simulink model "scd3busMicrogridDroopControlFidelityLevels3Inv"  (R2025b)
settings: Solver=ode15s  StartTime=0.0  StopTime=24  RelTol=1e-3
PreLoadFcn:
  | scd3busMicrogridDroopControlDataFidelityLevels3Inv;
  | 
  | %% Controller variants
  | % Create variant controls for converter controller. Controller has two
  | % different levels of fidelity: Averaged, AveragedPulse, Pulse
  | Averaged = Simulink.VariantExpression;
  | Averaged.Condition = 'fidelity==scd3busMicrogridDroopControl_variants_enum.Low';
  | Pulse = Simulink.VariantExpression;
  | Pulse.Condition = 'fidelity==scd3busMicrogridDroopControl_variants_enum.High';
  | 
  | %% Plant variants
  | % Create variant controls for converter plant. Plant has three different
  | % levels of fidelity.
  | AveragedNonSwitch = Simulink.VariantExpression;
  | AveragedNonSwitch.Condition = 'fidelity==scd3busMicrogridDroopControl_variants_enum.Low';
  | PulseSwitch = Simulink.VariantExpression;
  | PulseSwitch.Condition = 'fidelity==scd3busMicrogridDroopControl_variants_enum.High';
  | 
  | %% Set up variables ready for simulation
  | fidelity = scd3busMicrogridDroopControl_variants_enum.High;
  | Ts = 5e-6;
  | Ts_V = 1e-6;
  | Tsc = 1e-4;
  | Tsc_V = 5e-4;
values from neighbouring files (symbols this model uses):
  consensus_enable = 1    [scd3busMicrogridDroopControlDataFidelityLevels3Inv.m]
  fgrid = 60    [scd3busMicrogridDroopControlDataFidelityLevels.m]    (also in scd3busMicrogridDroopControlDataFidelityLevels3Inv.m)
  Kdroop_fp1 = 0.03/2    (= 0.015)    [scd3busMicrogridDroopControlDataFidelityLevels3Inv.m]
  Kdroop_fp2 = 0.03/2    (= 0.015)    [scd3busMicrogridDroopControlDataFidelityLevels3Inv.m]
  Kdroop_vq1 = 0.05/2    (= 0.025)    [scd3busMicrogridDroopControlDataFidelityLevels3Inv.m]
  Kdroop_vq2 = 0.05/2    (= 0.025)    [scd3busMicrogridDroopControlDataFidelityLevels3Inv.m]
  Ki_vd = 850    [scd3busMicrogridDroopControlDataFidelityLevels.m]    (also in scd3busMicrogridDroopControlDataFidelityLevels3Inv.m)
  Ki_vq = 850    [scd3busMicrogridDroopControlDataFidelityLevels.m]    (also in scd3busMicrogridDroopControlDataFidelityLevels3Inv.m)
  Kp_vd = 0.36    [scd3busMicrogridDroopControlDataFidelityLevels.m]    (also in scd3busMicrogridDroopControlDataFidelityLevels3Inv.m)
  Kp_vq = 0.36    [scd3busMicrogridDroopControlDataFidelityLevels.m]    (also in scd3busMicrogridDroopControlDataFidelityLevels3Inv.m)
  Vdc1 = 1000    [scd3busMicrogridDroopControlDataFidelityLevels.m]    (also in scd3busMicrogridDroopControlDataFidelityLevels3Inv.m)
  Vdc2 = 1000    [scd3busMicrogridDroopControlDataFidelityLevels.m]    (also in scd3busMicrogridDroopControlDataFidelityLevels3Inv.m)
  Vrms = 380    [scd3busMicrogridDroopControlDataFidelityLevels.m]    (also in scd3busMicrogridDroopControlDataFidelityLevels3Inv.m)
undefined symbols (not defined in the file or in its folder): DiscIntNeverNeededParam
libraries: ee_lib x29, nesl_utility x27, fl_lib x15, eeTransforms x4, eeSinusoidalMeasurement x4, slpidlib x4, eePwmGeneratorTwoLevel x2, eePowerMeasurement x2, simulink x2, SignalEditorBlockLib x1
(part 2 of 3)

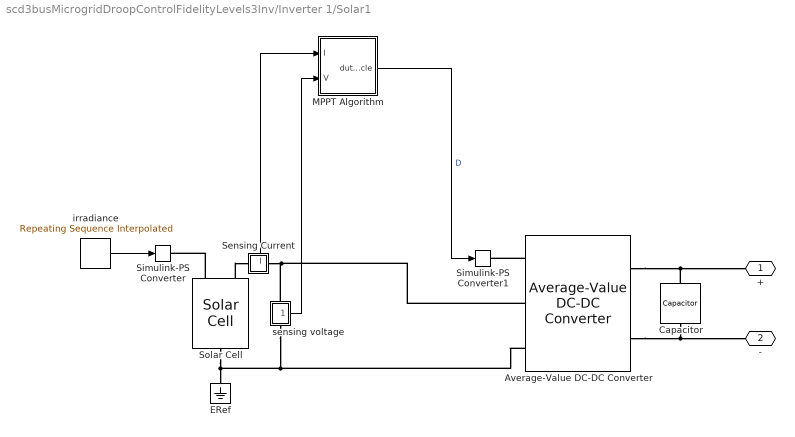
== system scd3busMicrogridDroopControlFidelityLevels3Inv/Inverter 1/Solar1 ==
  Average-Value DC-DC Converter : ee_lib/Semiconductors & Converters/Converters/Average-Value DC-DC Converter  implementation_option=ee.enum.converters.implementation.behavioral  converter_type=ee.enum.converters.dcdctype.boost  control_option=ee.enum.converters.controlinput.dutycycle  efficiency_option=ee.enum.converters.efficiency.constant  efficiency_fixed=100  i_vec=[0, 2, 5] A  efficiency_vec=[90, 95, 98]  Lf=1e-6 H  Rl=0 Ohm  Cf=1e-7 F  Rc=1e-6 Ohm  iL_specify=off  iL_priority=High  iL=0 A  iL_nominal_specify=off  iL_nominal_value=1  iL_nominal_unit=A  vc_specify=off  vc_priority=High  vc=0 V  vc_nominal_specify=off  vc_nominal_value=1  vc_nominal_unit=V
      settings: InternalSimscapePortConfiguration="{\"Bottom\":[],\"Left\":[{\"id\":\"DutyCycle\",\"label\":\"DutyCycle\",\"type\":\"input\"},{\"id\":\"p1\",\"label\":\"1+\",\"type\":\"foundation.electrical.electrical\"},{\"id\":\"n1\",\"label\":\"1-\",\"type\":\"foundation.electrical.electrical\"}],\"Right\":[{\"id\":\"p2\",\"label\":\"2+\",\"type\":\"foundation.electrical.electrical\"},{\"id\":\"n2\",\"label\":\"2-\",\"type\":\"foundation.electrical.electrical\"}],\"Top\":[]}"
  Capacitor : fl_lib/Electrical/Electrical Elements/Capacitor  c=10 mF  r=1e-6 Ohm  g=0 1/Ohm  i_specify=off  i_priority=None  i=0 A  i_nominal_specify=off  i_nominal_value=1  i_nominal_unit=A  v_specify=off  v_priority=None  v=0 V  v_nominal_specify=off  v_nominal_value=1  v_nominal_unit=V  vc_specify=off  vc_priority=High  vc=1000 V  vc_nominal_specify=off  vc_nominal_value=1  vc_nominal_unit=V
  ERef : fl_lib/Electrical/Electrical Elements/Electrical Reference
  MPPT Algorithm : Subsystem
  Sensing Current : Subsystem
      settings: PortSchema="{\"entries\":[{\"content\":{\"sides\":[{\"content\":{\"connectorIds\":[\"LConn1\"]},\"type\":\"ConnectorPlacement.EquallySpacedRectSide\",\"uuid\":\"08eaf192-3836-4d70-9f6a-c3aee0977ea6\"},{\"content\":{\"connectorIds\":[\"RConn1\"],\"side\":\"RIGHT\"},\"type\":\"ConnectorPlacement.EquallySpacedRectSide\",\"uuid\":\"69615d36-c1bf-4d31-b3e4-77c73286e7c7\"},{\"content\":{\"connectorIds\":[\"Out1\"],\"side\":\"TOP\"},\"type\":\"ConnectorPlacement.EquallySpacedRectSide\",\"uuid\":\"21e31d90-f675-47e5-98f5-1bf7e6a5fdbe\"}]},\"type\":\"ConnectorPlacement.EquallySpacedConnector\",\"uuid\":\"068abd2e-abc9-41d7-b40e-d83d3e3b9346\"}],\"packageUris\":[\"http://schema.mathworks.com/mf0/Connector/R2020b\"],\"version\":\"1.0\"}"
      mask Display: disp('i')
  Simulink-PS Converter : nesl_utility/Simulink-PS Converter  PhysicalDomain=network_engine_domain  SubClassName=ps_input  LeftPortType=input  RightPortType=output  PseudoPeriodic=off  Frequencies=[]  NoiseDistribution=none  NoiseParameters=[]  Unit=1  AffineConversion=off  FilteringAndDerivatives=provide  SimscapeFilterOrder=1  InputFilterTimeConstant=0.001  UdotUserProvided=0
  Simulink-PS Converter1 : nesl_utility/Simulink-PS Converter  PhysicalDomain=network_engine_domain  SubClassName=ps_input  LeftPortType=input  RightPortType=output  PseudoPeriodic=off  Frequencies=[]  NoiseDistribution=none  NoiseParameters=[]  Unit=1  AffineConversion=off  FilteringAndDerivatives=provide  SimscapeFilterOrder=1  InputFilterTimeConstant=0.001  UdotUserProvided=0
  Solar Cell : ee_lib/Sources/Solar Cell  prm=3  Isc=10.14 A  Voc=0.67 V  Is=3.24823447983853e-07 A  Is2=9.37081970792037e-10 A  Iph=10.140005507508 A  Ir0=1000 W/m^2  ec=1.51118472243322  N2=2.60259908345858  Rs=1.94548269975201e-05 Ohm  Rp=682.95993142779 Ohm  N_series=60 * 30  N_parallel=8  TIPH1=0.000499942933005141 1/K  EG=1.12 eV  TXIS1=4.23641510120988  TXIS2=16.2689137700667  TRS1=0.243341028305912  TRP1=0 % Parameter not set  Tmeas=25 degC  TFIXED=25 degC  thermal_mass=100 % Parameter not set J/K  initial_temperature=25 degC
  "irradiance " : simulink/Sources/Repeating Sequence Interpolated  OutValues=[5 5 5 5 5 5 5 5 5 5 5 5 5 5 5 5 5 5 5 5 5 5 5 5]*200  TimeValues=[0 1 2 3 4 5 6 7 8 9 10 11 12 13 14 15 16 17 18 19 20 21 22 23]  LookUpMeth=Interpolation-Use End Values  tsamp=Ts_DC  OutMin=[]  OutMax=[]  OutDataTypeStr=double  OutputDataTypeScalingMode=double  OutDataType=fixdt(0,8)  OutScaling=2^-10
  sensing voltage : Subsystem
      settings: PortSchema="{\"entries\":[{\"content\":{\"sides\":[{\"content\":{\"connectorIds\":[\"LConn1\"]},\"type\":\"ConnectorPlacement.EquallySpacedRectSide\",\"uuid\":\"08eaf192-3836-4d70-9f6a-c3aee0977ea6\"},{\"content\":{\"connectorIds\":[\"RConn1\"],\"side\":\"RIGHT\"},\"type\":\"ConnectorPlacement.EquallySpacedRectSide\",\"uuid\":\"69615d36-c1bf-4d31-b3e4-77c73286e7c7\"},{\"content\":{\"connectorIds\":[],\"side\":\"TOP\"},\"type\":\"ConnectorPlacement.EquallySpacedRectSide\",\"uuid\":\"21e31d90-f675-47e5-98f5-1bf7e6a5fdbe\"},{\"content\":{\"connectorIds\":[\"Out1\"],\"side\":\"BOTTOM\"},\"type\":\"ConnectorPlacement.EquallySpacedRectSide\",\"uuid\":\"23a77980-6beb-4147-b48e-adf9e1983263\"}]},\"type\":\"ConnectorPlacement.EquallySpacedConnector\",\"uuid\":\"068abd2e-abc9-41d7-b40e-d83d3e3b9346\"}],\"packageUris\":[\"http://schema.mathworks.com/mf0/Connector/R2020b\"],\"version\":\"1.0\"}"
      mask Display: disp('v')
  + : PMIOPort  Side=Right
  - : PMIOPort  Port=2  Side=Right
  wires:
  "irradiance "/1 -> Simulink-PS Converter/1
  Sensing Current/1(I) -> MPPT Algorithm/1(I)
  sensing voltage/1(V) -> MPPT Algorithm/2(V)
  MPPT Algorithm/1(duty_cycle) -> Simulink-PS Converter1/1  "D"
  connections:
  Average-Value DC-DC Converter/LConn2 -- Sensing Current/RConn1 -- sensing voltage/LConn1
  Average-Value DC-DC Converter/LConn3 -- sensing voltage/RConn1 -- ERef/LConn1 -- Solar Cell/RConn1
  Average-Value DC-DC Converter/LConn1 -- Simulink-PS Converter1/RConn1
  Solar Cell/LConn1 -- Simulink-PS Converter/RConn1
  Solar Cell/LConn2 -- Sensing Current/LConn1
  Average-Value DC-DC Converter/RConn1 -- +/RConn1 -- Capacitor/LConn1
  Average-Value DC-DC Converter/RConn2 -- -/RConn1 -- Capacitor/RConn1

== system scd3busMicrogridDroopControlFidelityLevels3Inv/Inverter 2/Average-Value Signal1 ==
  ModWave : Inport
  Bias : Bias  Bias=1  SaturateOnIntegerOverflow=off
  Bias1 : Bias  Bias=1  SaturateOnIntegerOverflow=off
  Gain : Gain  Gain=-1
  Mod. Index1 : Gain  Gain=0.5
  Mux : Mux  Inputs=2
  Rate Transition : RateTransition  OutPortSampleTime=Ts_V
  Selector4 : Selector  InputPortWidth=6  IndexOptions=Index vector (dialog)  Indices=[1 4 2 5 3 6]  OutputSizes=1
  DutyCycle : Outport
  wires:
  ModWave/1 -> Rate Transition/1
  Gain/1 -> Bias1/1
  Mod. Index1/1 -> Gain/1, Mux/1
  Bias/1 -> Mod. Index1/1
  Rate Transition/1 -> Bias/1
  Selector4/1 -> DutyCycle/1
  Bias1/1 -> Mux/2
  Mux/1 -> Selector4/1

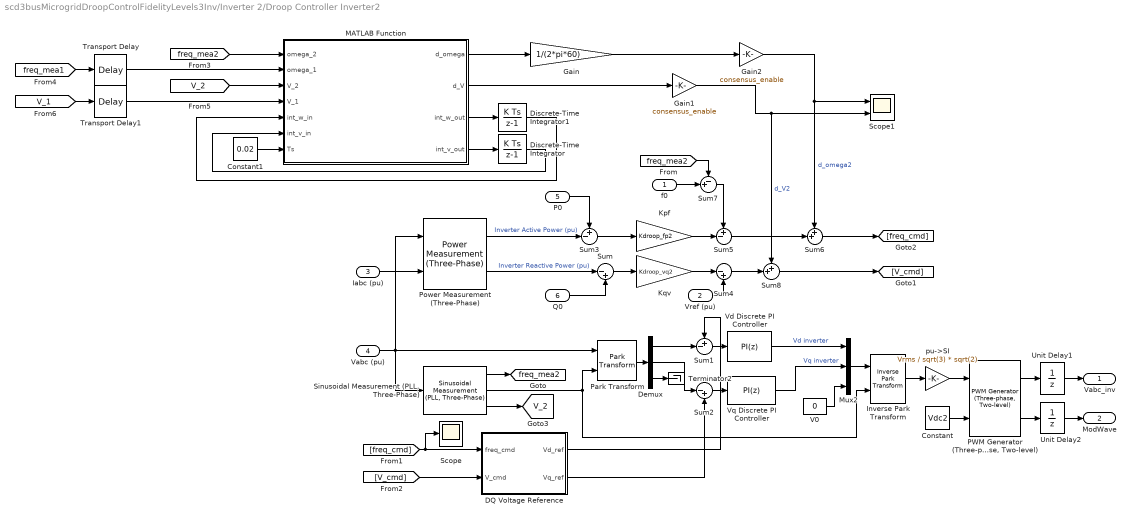
== system scd3busMicrogridDroopControlFidelityLevels3Inv/Inverter 2/Droop Controller Inverter2 ==
  f0 : Inport
  Vref (pu) : Inport  Port=2
  Iabc (pu) : Inport  Port=3
  Vabc (pu) : Inport  Port=4
  P0 : Inport  Port=5
  Q0 : Inport  Port=6
  Constant : Constant  Value=Vdc2
  Constant1 : Constant  Value=0.02
  DQ Voltage Reference : Subsystem
  Demux : Demux  Outputs=3
  Discrete-Time Integrator : DiscreteIntegrator  SampleTime=0.02  ICPrevOutput=DiscIntNeverNeededParam  ICPrevScaledInput=DiscIntNeverNeededParam
  Discrete-Time Integrator1 : DiscreteIntegrator  SampleTime=0.02  ICPrevOutput=DiscIntNeverNeededParam  ICPrevScaledInput=DiscIntNeverNeededParam
  Gain : Gain  Gain=1/(2*pi*60)
  Gain1 : Gain  Gain=consensus_enable
  Gain2 : Gain  Gain=consensus_enable
  Inverse Park Transform : eeTransforms/Inverse Park Transform  AxisAlignment=Q-axis  PowerInvariant=off
  Kpf : Gain  Gain=Kdroop_fp2
  Kqv : Gain  Gain=Kdroop_vq2
  MATLAB Function : MATLAB Function  TreatAsAtomicUnit=on
  Mux2 : Mux  Inputs=3
  "PWM Generator (Three-phase, Two-level)" : eePwmGeneratorTwoLevel/PWM Generator (Three-phase, Two-level)  PWMMode=Continuous PWM (CPWM)  CPWMMode=SPWM: sinusoidal PWM  DPWMMode=60 DPWM: 60 degree discontinuous PWM  fsw=fsw_V  Ts=Ts_V
  Park Transform : eeTransforms/Park Transform  AxisAlignment=Q-axis  PowerInvariant=off
  Power Measurement (Three-Phase) : eePowerMeasurement/Power Measurement (Three-Phase)  LabelModeActiveChoice=Discrete  F=fgrid  K=1  Seq=Positive  Ts=Ts
  Scope : Scope
      settings: ActiveDisplayYMinimum=-2.22443  ActiveDisplayYMaximum=1.7851
  Scope1 : Scope  NumInputPorts=2
      settings: ActiveDisplayYMinimum=-0.013262911924324612  ActiveDisplayYMaximum=0.013262911924324612
  "Sinusoidal Measurement (PLL, Three-Phase)" : eeSinusoidalMeasurement/Sinusoidal Measurement (PLL, Three-Phase)  Kp_LF=180  Ki_LF=3200  F0=fgrid  Theta0=0  Ts=Ts_V
  Sum : Sum  Inputs=|-+
  Sum1 : Sum  Inputs=+-|  InputSameDT=on  SaturateOnIntegerOverflow=on  OutDataTypeStr=Inherit: Same as first input
  Sum2 : Sum  Inputs=|-+  InputSameDT=on  SaturateOnIntegerOverflow=on  OutDataTypeStr=Inherit: Same as first input
  Sum3 : Sum  Inputs=+-|
  Sum4 : Sum  Inputs=|-+
  Sum5 : Sum  Inputs=+-|
  Sum6 : Sum  Inputs=++|
  Sum7 : Sum  Inputs=-+|
  Sum8 : Sum  Inputs=++|
  Terminator2 : Terminator
  Transport Delay : TransportDelay  DelayTime=0.1
  Transport Delay1 : TransportDelay  DelayTime=0.1
  Unit Delay1 : UnitDelay  SampleTime=Ts_V  HasFrameUpgradeWarning=on
  Unit Delay2 : UnitDelay  SampleTime=Ts_V  HasFrameUpgradeWarning=on
  V0 : Constant  Value=0
  Vd Discrete PI Controller : slpidlib/PID Controller  Controller=PI  Form=Parallel  TimeDomain=Discrete-time  UseExternalTs=off  SampleTime=Ts_V  IntegratorMethod=Forward Euler  FilterMethod=Forward Euler  ControllerParametersSource=internal  P=Kp_vd  I=Ki_vd  UseKiTs=off  D=0  UseExternalDerivativeSource=off  N=100  UseFilter=on  TunerSelectOption=Transfer Function Based (PID Tuner App)  InitialConditionSource=internal  InitialConditionForIntegrator=0.62  InitialConditionForFilter=0  DifferentiatorICPrevScaledInput=0  ExternalReset=none  TrackingMode=off  Kt=1  LimitOutput=on  SatLimitsSource=internal  UpperSaturationLimit=1  LowerSaturationLimit=0  LinearizeAsGain=on  AntiWindupMode=none  Kb=1  LimitIntegrator=off  UpperIntegratorSaturationLimit=inf  LowerIntegratorSaturationLimit=-inf  POutMin=[]  POutMax=[]  IOutMin=[]  IOutMax=[]  DOutMin=[]  DOutMax=[]  NOutMin=[]  NOutMax=[]  SumOutMin=[]  SumOutMax=[]  SaturationOutMin=[]  SaturationOutMax=[]  PParamMin=[]  PParamMax=[]  IParamMin=[]  IParamMax=[]  DParamMin=[]  DParamMax=[]  NParamMin=[]  NParamMax=[]  KbParamMin=[]  KbParamMax=[]  KtParamMin=[]  KtParamMax=[]  KbOutMin=[]  KbOutMax=[]  KtOutMin=[]  KtOutMax=[]  IntegratorOutMin=[]  IntegratorOutMax=[]  FilterOutMin=[]  FilterOutMax=[]  SumI1OutMin=[]  SumI1OutMax=[]  SumI2OutMin=[]  SumI2OutMax=[]  SumI3OutMin=[]  SumI3OutMax=[]  SumI4OutMin=[]  SumI4OutMax=[]  SumDOutMin=[]  SumDOutMax=[]  DifferentiatorOutMin=[]  DifferentiatorOutMax=[]  FilterDiffOutCoefMin=[]  FilterDiffOutCoefMax=[]  ReciprocalOutMin=[]  ReciprocalOutMax=[]  SumDenOutMin=[]  SumDenOutMax=[]  SumNumOutMin=[]  SumNumOutMax=[]  DivideOutMin=[]  DivideOutMax=[]  UdiffTsProdOutMin=[]  UdiffTsProdOutMax=[]  NTsProdOutMin=[]  NTsProdOutMax=[]  UintegralTsProdOutMin=[]  UintegralTsProdOutMax=[]  UngainTsProdOutMin=[]  UngainTsProdOutMax=[]  ClampingZeroOutDataTypeStr=Inherit: Inherit via back propagation  ClampingZeroOutMin=[]  ClampingZeroOutMax=[]  FilterDenConstantOutDataTypeStr=Inherit: Inherit via back propagation  FilterDenConstantOutMin=[]  FilterDenConstantOutMax=[]  PCopyOutDataTypeStr=Inherit: Inherit via back propagation  PCopyOutMin=[]  PCopyOutMax=[]  NCopyOutDataTypeStr=Inherit: Inherit via back propagation  NCopyOutMin=[]  NCopyOutMax=[]  IntegratorContinuousStateAttributes=''  IntegratorStateMustResolveToSignalObject=off  IntegratorRTWStateStorageClass=Auto  FilterContinuousStateAttributes=''  FilterStateMustResolveToSignalObject=off  FilterRTWStateStorageClass=Auto  ParallelPVariant=InternalParameters  IdealPVariant=Disabled  IVariant=InternalParameters  DVariant=Disabled  IntegratorVariant=Discrete  SatVariant=Enabled  AWVariant=Passthrough  PCopyVariant=Disabled  TRVariant=Disabled  FdbkBlocksVariant=Forward  IdealPFdbkVariant=Disabled  SatFdbkVariant=Disabled  DerivativeFilterVariant=Disabled  NVariant=Disabled  NCopyVariant=Disabled_SignalSpec  FilterICVariant=Disabled  IntegratorICVariant=InternalICs  ExternalResetVariant=Disabled  TRSumVariant=Passthrough  SumFdbkVariant=Disabled  SumVariant=Sum_PI  TsampFilterVariant=InternalTs  TsampNgainVariant=Passthrough  TsampIntegralVariant=Disabled_SignalSpec  ExternalSaturationOutDataTypeStr=Inherit: Same as second input  DerivativeSourceVariant=Disabled  PreIntVariant=InternalPreInt
  Vq Discrete PI Controller : slpidlib/PID Controller  Controller=PI  Form=Parallel  TimeDomain=Discrete-time  UseExternalTs=off  SampleTime=Ts_V  IntegratorMethod=Forward Euler  FilterMethod=Forward Euler  ControllerParametersSource=internal  P=Kp_vq  I=Ki_vq  UseKiTs=off  D=0  UseExternalDerivativeSource=off  N=100  UseFilter=on  TunerSelectOption=Transfer Function Based (PID Tuner App)  InitialConditionSource=internal  InitialConditionForIntegrator=0  InitialConditionForFilter=0  DifferentiatorICPrevScaledInput=0  ExternalReset=none  TrackingMode=off  Kt=1  LimitOutput=on  SatLimitsSource=internal  UpperSaturationLimit=1  LowerSaturationLimit=0  LinearizeAsGain=on  AntiWindupMode=none  Kb=1  LimitIntegrator=off  UpperIntegratorSaturationLimit=inf  LowerIntegratorSaturationLimit=-inf  POutMin=[]  POutMax=[]  IOutMin=[]  IOutMax=[]  DOutMin=[]  DOutMax=[]  NOutMin=[]  NOutMax=[]  SumOutMin=[]  SumOutMax=[]  SaturationOutMin=[]  SaturationOutMax=[]  PParamMin=[]  PParamMax=[]  IParamMin=[]  IParamMax=[]  DParamMin=[]  DParamMax=[]  NParamMin=[]  NParamMax=[]  KbParamMin=[]  KbParamMax=[]  KtParamMin=[]  KtParamMax=[]  KbOutMin=[]  KbOutMax=[]  KtOutMin=[]  KtOutMax=[]  IntegratorOutMin=[]  IntegratorOutMax=[]  FilterOutMin=[]  FilterOutMax=[]  SumI1OutMin=[]  SumI1OutMax=[]  SumI2OutMin=[]  SumI2OutMax=[]  SumI3OutMin=[]  SumI3OutMax=[]  SumI4OutMin=[]  SumI4OutMax=[]  SumDOutMin=[]  SumDOutMax=[]  DifferentiatorOutMin=[]  DifferentiatorOutMax=[]  FilterDiffOutCoefMin=[]  FilterDiffOutCoefMax=[]  ReciprocalOutMin=[]  ReciprocalOutMax=[]  SumDenOutMin=[]  SumDenOutMax=[]  SumNumOutMin=[]  SumNumOutMax=[]  DivideOutMin=[]  DivideOutMax=[]  UdiffTsProdOutMin=[]  UdiffTsProdOutMax=[]  NTsProdOutMin=[]  NTsProdOutMax=[]  UintegralTsProdOutMin=[]  UintegralTsProdOutMax=[]  UngainTsProdOutMin=[]  UngainTsProdOutMax=[]  ClampingZeroOutDataTypeStr=Inherit: Inherit via back propagation  ClampingZeroOutMin=[]  ClampingZeroOutMax=[]  FilterDenConstantOutDataTypeStr=Inherit: Inherit via back propagation  FilterDenConstantOutMin=[]  FilterDenConstantOutMax=[]  PCopyOutDataTypeStr=Inherit: Inherit via back propagation  PCopyOutMin=[]  PCopyOutMax=[]  NCopyOutDataTypeStr=Inherit: Inherit via back propagation  NCopyOutMin=[]  NCopyOutMax=[]  IntegratorContinuousStateAttributes=''  IntegratorStateMustResolveToSignalObject=off  IntegratorRTWStateStorageClass=Auto  FilterContinuousStateAttributes=''  FilterStateMustResolveToSignalObject=off  FilterRTWStateStorageClass=Auto  ParallelPVariant=InternalParameters  IdealPVariant=Disabled  IVariant=InternalParameters  DVariant=Disabled  IntegratorVariant=Discrete  SatVariant=Enabled  AWVariant=Passthrough  PCopyVariant=Disabled  TRVariant=Disabled  FdbkBlocksVariant=Forward  IdealPFdbkVariant=Disabled  SatFdbkVariant=Disabled  DerivativeFilterVariant=Disabled  NVariant=Disabled  NCopyVariant=Disabled_SignalSpec  FilterICVariant=Disabled  IntegratorICVariant=InternalICs  ExternalResetVariant=Disabled  TRSumVariant=Passthrough  SumFdbkVariant=Disabled  SumVariant=Sum_PI  TsampFilterVariant=InternalTs  TsampNgainVariant=Passthrough  TsampIntegralVariant=Disabled_SignalSpec  ExternalSaturationOutDataTypeStr=Inherit: Same as second input  DerivativeSourceVariant=Disabled  PreIntVariant=InternalPreInt
  pu->SI : Gain  Gain=Vrms / sqrt(3) * sqrt(2)
  Vabc_inv : Outport
  ModWave : Outport  Port=2
  tag scope: V_2=global, freq_mea2=global
  wires:
  DQ Voltage Reference/2(Vq_ref) -> Sum2/2
  [V_cmd] -> DQ Voltage Reference/2(V_cmd)
  [freq_cmd] -> Scope/1, DQ Voltage Reference/1(freq_cmd)
  Sum4/1 -> Sum8/2
  Sum5/1 -> Sum6/2
  [freq_mea2] -> Sum7/1
  Sum7/1 -> Sum5/1
  Vref (pu)/1 -> Sum4/2
  f0/1 -> Sum7/2
  Kqv/1 -> Sum4/1
  Kpf/1 -> Sum5/2
  Sum3/1 -> Kpf/1
  Sum/1 -> Kqv/1
  Q0/1 -> Sum/2
  P0/1 -> Sum3/1
  Power Measurement (Three-Phase)/2 -> Sum/1  "Inverter Reactive Power (pu)"
  Power Measurement (Three-Phase)/1 -> Sum3/2  "Inverter Active Power (pu)"
  Iabc (pu)/1 -> Power Measurement (Three-Phase)/2
  Vabc (pu)/1 -> Park Transform/1, "Sinusoidal Measurement (PLL, Three-Phase)"/1, Power Measurement (Three-Phase)/1
  pu->SI/1 -> "PWM Generator (Three-phase, Two-level)"/1
  Unit Delay1/1 -> Vabc_inv/1
  "PWM Generator (Three-phase, Two-level)"/2 -> Unit Delay2/1
  "PWM Generator (Three-phase, Two-level)"/1 -> Unit Delay1/1
  Inverse Park Transform/1 -> pu->SI/1
  Constant/1 -> "PWM Generator (Three-phase, Two-level)"/2
  "Sinusoidal Measurement (PLL, Three-Phase)"/1 -> [freq_mea2]
  "Sinusoidal Measurement (PLL, Three-Phase)"/2 -> Park Transform/2, Inverse Park Transform/2
  "Sinusoidal Measurement (PLL, Three-Phase)"/3 -> [V_2]
  Demux/3 -> Terminator2/1
  Demux/1 -> Sum1/2
  V0/1 -> Mux2/3
  Vq Discrete PI Controller/1 -> Mux2/2  "Vq inverter"
  Demux/2 -> Sum2/1
  Sum2/1 -> Vq Discrete PI Controller/1
  Park Transform/1 -> Demux/1
  Sum1/1 -> Vd Discrete PI Controller/1
  Mux2/1 -> Inverse Park Transform/1
  Vd Discrete PI Controller/1 -> Mux2/1  "Vd inverter"
  DQ Voltage Reference/1(Vd_ref) -> Sum1/1
  Unit Delay2/1 -> ModWave/1
  [freq_mea2] -> MATLAB Function/1(omega_2)
  [freq_mea1] -> Transport Delay/1
  [V_2] -> MATLAB Function/3(V_2)
  MATLAB Function/4(int_v_out) -> Discrete-Time Integrator/1
  MATLAB Function/3(int_w_out) -> Discrete-Time Integrator1/1
  Discrete-Time Integrator/1 -> MATLAB Function/6(int_v_in)
  Discrete-Time Integrator1/1 -> MATLAB Function/5(int_w_in)
  Constant1/1 -> MATLAB Function/7(Ts)
  MATLAB Function/1(d_omega) -> Gain/1
  Sum6/1 -> [freq_cmd]
  Gain/1 -> Gain2/1
  MATLAB Function/2(d_V) -> Gain1/1
  Sum8/1 -> [V_cmd]
  Transport Delay/1 -> MATLAB Function/2(omega_1)
  [V_1] -> Transport Delay1/1
  Transport Delay1/1 -> MATLAB Function/4(V_1)
  Gain1/1 -> Sum8/1, Scope1/2  "d_V2"
  Gain2/1 -> Sum6/1, Scope1/1  "d_omega2"

== system scd3busMicrogridDroopControlFidelityLevels3Inv/Inverter 2/Gate driver1 ==
  DutyCycle : Inport
  Data Type Conversion : DataTypeConversion  SaturateOnIntegerOverflow=off  RndMeth=Floor
  Demux : Demux  Outputs=6
  Simulink-PS Converter{,1..5} (6 alike) : nesl_utility/Simulink-PS Converter  PhysicalDomain=network_engine_domain  SubClassName=ps_input  LeftPortType=input  RightPortType=output  PseudoPeriodic=off  Frequencies=[]  NoiseDistribution=none  NoiseParameters=[]  Unit=1  AffineConversion=off  FilteringAndDerivatives=provide  SimscapeFilterOrder=1  InputFilterTimeConstant=0.001  UdotUserProvided=0
  Six-Pulse Gate Multiplexer : ee_lib/Semiconductors & Converters/Converters/Six-Pulse Gate Multiplexer  port_option=ee.enum.controlport.ps
  G : PMIOPort  Side=Right
  wires:
  Demux/5 -> Simulink-PS Converter4/1
  Demux/3 -> Simulink-PS Converter2/1
  Data Type Conversion/1 -> Demux/1
  Demux/4 -> Simulink-PS Converter3/1
  Demux/6 -> Simulink-PS Converter5/1
  Demux/2 -> Simulink-PS Converter1/1
  Demux/1 -> Simulink-PS Converter/1
  DutyCycle/1 -> Data Type Conversion/1
  connections:
  Simulink-PS Converter4/RConn1 -- Six-Pulse Gate Multiplexer/LConn5
  Simulink-PS Converter2/RConn1 -- Six-Pulse Gate Multiplexer/LConn3
  Simulink-PS Converter/RConn1 -- Six-Pulse Gate Multiplexer/LConn1
  Simulink-PS Converter5/RConn1 -- Six-Pulse Gate Multiplexer/LConn6
  Simulink-PS Converter1/RConn1 -- Six-Pulse Gate Multiplexer/LConn2
  Simulink-PS Converter3/RConn1 -- Six-Pulse Gate Multiplexer/LConn4
  Six-Pulse Gate Multiplexer/RConn1 -- G/RConn1

== system scd3busMicrogridDroopControlFidelityLevels3Inv/Inverter 2/Inverter 2 ==
  Averaged Inverter : Subsystem  VariantControl=AveragedNonSwitch
  IGBT Inverter : Subsystem  VariantControl=PulseSwitch
  + : PMIOPort  Side=Right
  G : PMIOPort  Port=2  Side=Left
  a : PMIOPort  Port=3  Side=Left
  b : PMIOPort  Port=4  Side=Left
  - : PMIOPort  Port=5  Side=Right
  c : PMIOPort  Port=6  Side=Left

== system scd3busMicrogridDroopControlFidelityLevels3Inv/Inverter 2/Measurement inverter1 ==
  Current and Voltage Sensor (Three-Phase) : ee_lib/Sensors & Transducers/Current and Voltage Sensor (Three-Phase)  vMeasurementType=ee.enum.vmeasurement.lg  outputUnit=ee.enum.unit.pu  SRated=150000 A*V  VRated=Vrms V  I_specify=off  I_priority=None  I=[ 0 0 0 ] A  I_nominal_specify=off  I_nominal_value=1  I_nominal_unit=A  V_specify=off  V_priority=None  V=[ 0 0 0 ] V  V_nominal_specify=off  V_nominal_value=1  V_nominal_unit=V
      settings: InternalSimscapePortConfiguration="{\"Bottom\":[],\"Left\":[{\"id\":\"a1\",\"label\":\"a1\",\"type\":\"foundation.electrical.electrical\"},{\"id\":\"b1\",\"label\":\"b1\",\"type\":\"foundation.electrical.electrical\"},{\"id\":\"c1\",\"label\":\"c1\",\"type\":\"foundation.electrical.electrical\"}],\"Right\":[{\"id\":\"V_output\",\"label\":\"V\",\"type\":\"output\"},{\"id\":\"I_output\",\"label\":\"I\",\"type\":\"output\"},{\"id\":\"a2\",\"label\":\"a2\",\"type\":\"foundation.electrical.electrical\"},{\"id\":\"b2\",\"label\":\"b2\",\"type\":\"foundation.electrical.electrical\"},{\"id\":\"c2\",\"label\":\"c2\",\"type\":\"foundation.electrical.electrical\"}],\"Top\":[]}"
  PS-Simulink Converter2 : nesl_utility/PS-Simulink Converter  PhysicalDomain=network_engine_domain  SubClassName=ps_output  LeftPortType=input  RightPortType=output  PseudoPeriodic=off  Frequencies=[]  VectorFormat=1-D array  Unit=1  AffineConversion=off
  PS-Simulink Converter3 : nesl_utility/PS-Simulink Converter  PhysicalDomain=network_engine_domain  SubClassName=ps_output  LeftPortType=input  RightPortType=output  PseudoPeriodic=off  Frequencies=[]  VectorFormat=1-D array  Unit=1  AffineConversion=off
  a1 : PMIOPort  Side=Left
  b1 : PMIOPort  Port=2  Side=Left
  a2 : PMIOPort  Port=3  Side=Right
  b2 : PMIOPort  Port=4  Side=Right
  c1 : PMIOPort  Port=5  Side=Left
  c2 : PMIOPort  Port=6  Side=Right
  tag scope: Iabc_inverter2=global, Vabc_inverter2=global
  wires:
  PS-Simulink Converter2/1 -> [Vabc_inverter2]
  PS-Simulink Converter3/1 -> [Iabc_inverter2]
  connections:
  b2/RConn1 -- Current and Voltage Sensor (Three-Phase)/RConn4
  a2/RConn1 -- Current and Voltage Sensor (Three-Phase)/RConn3
  Current and Voltage Sensor (Three-Phase)/RConn5 -- c2/RConn1
  Current and Voltage Sensor (Three-Phase)/LConn2 -- b1/RConn1
  Current and Voltage Sensor (Three-Phase)/LConn3 -- c1/RConn1
  Current and Voltage Sensor (Three-Phase)/LConn1 -- a1/RConn1
  PS-Simulink Converter2/LConn1 -- Current and Voltage Sensor (Three-Phase)/RConn1
  Current and Voltage Sensor (Three-Phase)/RConn2 -- PS-Simulink Converter3/LConn1

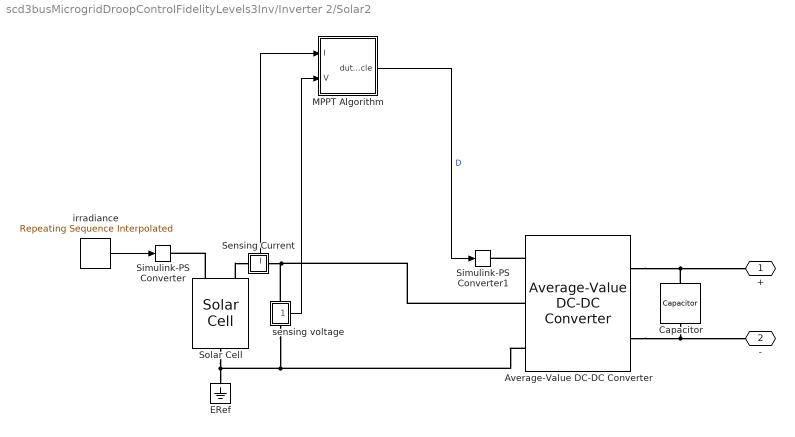
== system scd3busMicrogridDroopControlFidelityLevels3Inv/Inverter 2/Solar2 ==
  Average-Value DC-DC Converter : ee_lib/Semiconductors & Converters/Converters/Average-Value DC-DC Converter  implementation_option=ee.enum.converters.implementation.behavioral  converter_type=ee.enum.converters.dcdctype.boost  control_option=ee.enum.converters.controlinput.dutycycle  efficiency_option=ee.enum.converters.efficiency.constant  efficiency_fixed=100  i_vec=[0, 2, 5] A  efficiency_vec=[90, 95, 98]  Lf=1e-6 H  Rl=0 Ohm  Cf=1e-7 F  Rc=1e-6 Ohm  iL_specify=off  iL_priority=High  iL=0 A  iL_nominal_specify=off  iL_nominal_value=1  iL_nominal_unit=A  vc_specify=off  vc_priority=High  vc=0 V  vc_nominal_specify=off  vc_nominal_value=1  vc_nominal_unit=V
      settings: InternalSimscapePortConfiguration="{\"Bottom\":[],\"Left\":[{\"id\":\"DutyCycle\",\"label\":\"DutyCycle\",\"type\":\"input\"},{\"id\":\"p1\",\"label\":\"1+\",\"type\":\"foundation.electrical.electrical\"},{\"id\":\"n1\",\"label\":\"1-\",\"type\":\"foundation.electrical.electrical\"}],\"Right\":[{\"id\":\"p2\",\"label\":\"2+\",\"type\":\"foundation.electrical.electrical\"},{\"id\":\"n2\",\"label\":\"2-\",\"type\":\"foundation.electrical.electrical\"}],\"Top\":[]}"
  Capacitor : fl_lib/Electrical/Electrical Elements/Capacitor  c=10 mF  r=1e-6 Ohm  g=0 1/Ohm  i_specify=off  i_priority=None  i=0 A  i_nominal_specify=off  i_nominal_value=1  i_nominal_unit=A  v_specify=off  v_priority=None  v=0 V  v_nominal_specify=off  v_nominal_value=1  v_nominal_unit=V  vc_specify=off  vc_priority=High  vc=1000 V  vc_nominal_specify=off  vc_nominal_value=1  vc_nominal_unit=V
  ERef : fl_lib/Electrical/Electrical Elements/Electrical Reference
  MPPT Algorithm : Subsystem
  Sensing Current : Subsystem
      settings: PortSchema="{\"entries\":[{\"content\":{\"sides\":[{\"content\":{\"connectorIds\":[\"LConn1\"]},\"type\":\"ConnectorPlacement.EquallySpacedRectSide\",\"uuid\":\"08eaf192-3836-4d70-9f6a-c3aee0977ea6\"},{\"content\":{\"connectorIds\":[\"RConn1\"],\"side\":\"RIGHT\"},\"type\":\"ConnectorPlacement.EquallySpacedRectSide\",\"uuid\":\"69615d36-c1bf-4d31-b3e4-77c73286e7c7\"},{\"content\":{\"connectorIds\":[\"Out1\"],\"side\":\"TOP\"},\"type\":\"ConnectorPlacement.EquallySpacedRectSide\",\"uuid\":\"21e31d90-f675-47e5-98f5-1bf7e6a5fdbe\"}]},\"type\":\"ConnectorPlacement.EquallySpacedConnector\",\"uuid\":\"068abd2e-abc9-41d7-b40e-d83d3e3b9346\"}],\"packageUris\":[\"http://schema.mathworks.com/mf0/Connector/R2020b\"],\"version\":\"1.0\"}"
      mask Display: disp('i')
  Simulink-PS Converter : nesl_utility/Simulink-PS Converter  PhysicalDomain=network_engine_domain  SubClassName=ps_input  LeftPortType=input  RightPortType=output  PseudoPeriodic=off  Frequencies=[]  NoiseDistribution=none  NoiseParameters=[]  Unit=1  AffineConversion=off  FilteringAndDerivatives=provide  SimscapeFilterOrder=1  InputFilterTimeConstant=0.001  UdotUserProvided=0
  Simulink-PS Converter1 : nesl_utility/Simulink-PS Converter  PhysicalDomain=network_engine_domain  SubClassName=ps_input  LeftPortType=input  RightPortType=output  PseudoPeriodic=off  Frequencies=[]  NoiseDistribution=none  NoiseParameters=[]  Unit=1  AffineConversion=off  FilteringAndDerivatives=provide  SimscapeFilterOrder=1  InputFilterTimeConstant=0.001  UdotUserProvided=0
  Solar Cell : ee_lib/Sources/Solar Cell  prm=3  Isc=10.14 A  Voc=0.67 V  Is=3.24823447983853e-07 A  Is2=9.37081970792037e-10 A  Iph=10.140005507508 A  Ir0=1000 W/m^2  ec=1.51118472243322  N2=2.60259908345858  Rs=1.94548269975201e-05 Ohm  Rp=682.95993142779 Ohm  N_series=60 * 21  N_parallel=7  TIPH1=0.000499942933005141 1/K  EG=1.12 eV  TXIS1=4.23641510120988  TXIS2=16.2689137700667  TRS1=0.243341028305912  TRP1=0 % Parameter not set  Tmeas=25 degC  TFIXED=25 degC  thermal_mass=100 % Parameter not set J/K  initial_temperature=25 degC
  "irradiance " : simulink/Sources/Repeating Sequence Interpolated  OutValues=[5 5 5 5 5 5 5 5 5 5 5 5 5 5 5 5 5 5 5 5 5 5 5 5]*200  TimeValues=[0 1 2 3 4 5 6 7 8 9 10 11 12 13 14 15 16 17 18 19 20 21 22 23]  LookUpMeth=Interpolation-Use End Values  tsamp=Ts_DC  OutMin=[]  OutMax=[]  OutDataTypeStr=double  OutputDataTypeScalingMode=double  OutDataType=fixdt(0,8)  OutScaling=2^-10
  sensing voltage : Subsystem
      settings: PortSchema="{\"entries\":[{\"content\":{\"sides\":[{\"content\":{\"connectorIds\":[\"LConn1\"]},\"type\":\"ConnectorPlacement.EquallySpacedRectSide\",\"uuid\":\"08eaf192-3836-4d70-9f6a-c3aee0977ea6\"},{\"content\":{\"connectorIds\":[\"RConn1\"],\"side\":\"RIGHT\"},\"type\":\"ConnectorPlacement.EquallySpacedRectSide\",\"uuid\":\"69615d36-c1bf-4d31-b3e4-77c73286e7c7\"},{\"content\":{\"connectorIds\":[],\"side\":\"TOP\"},\"type\":\"ConnectorPlacement.EquallySpacedRectSide\",\"uuid\":\"21e31d90-f675-47e5-98f5-1bf7e6a5fdbe\"},{\"content\":{\"connectorIds\":[\"Out1\"],\"side\":\"BOTTOM\"},\"type\":\"ConnectorPlacement.EquallySpacedRectSide\",\"uuid\":\"23a77980-6beb-4147-b48e-adf9e1983263\"}]},\"type\":\"ConnectorPlacement.EquallySpacedConnector\",\"uuid\":\"068abd2e-abc9-41d7-b40e-d83d3e3b9346\"}],\"packageUris\":[\"http://schema.mathworks.com/mf0/Connector/R2020b\"],\"version\":\"1.0\"}"
      mask Display: disp('v')
  + : PMIOPort  Side=Right
  - : PMIOPort  Port=2  Side=Right
  wires:
  "irradiance "/1 -> Simulink-PS Converter/1
  Sensing Current/1(I) -> MPPT Algorithm/1(I)
  sensing voltage/1(V) -> MPPT Algorithm/2(V)
  MPPT Algorithm/1(duty_cycle) -> Simulink-PS Converter1/1  "D"
  connections:
  Average-Value DC-DC Converter/LConn2 -- Sensing Current/RConn1 -- sensing voltage/LConn1
  Average-Value DC-DC Converter/LConn3 -- sensing voltage/RConn1 -- Solar Cell/RConn1 -- ERef/LConn1
  Average-Value DC-DC Converter/LConn1 -- Simulink-PS Converter1/RConn1
  Solar Cell/LConn1 -- Simulink-PS Converter/RConn1
  Solar Cell/LConn2 -- Sensing Current/LConn1
  Average-Value DC-DC Converter/RConn1 -- +/RConn1 -- Capacitor/LConn1
  Average-Value DC-DC Converter/RConn2 -- -/RConn1 -- Capacitor/RConn1

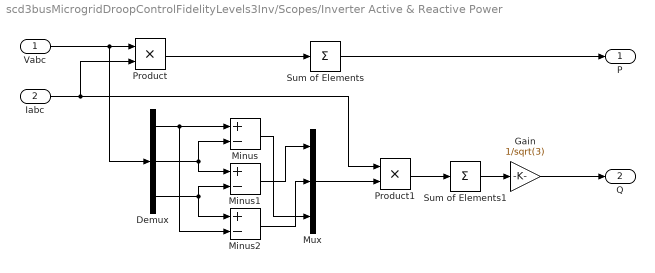
== system scd3busMicrogridDroopControlFidelityLevels3Inv/Scopes/Inverter Active & Reactive Power  ==
  Vabc : Inport
  Iabc : Inport  Port=2
  Demux : Demux  Outputs=3
  Gain : Gain  Gain=1/sqrt(3)
  Minus : Sum  Inputs=+-
  Minus1 : Sum  Inputs=+-
  Minus2 : Sum  Inputs=+-
  Mux : Mux  Inputs=3
  Product : Product
  Product1 : Product
  Sum of Elements : Sum  Inputs=+
  Sum of Elements1 : Sum  Inputs=+
  P : Outport  VectorParamsAs1DForOutWhenUnconnected=off
  Q : Outport  Port=2  VectorParamsAs1DForOutWhenUnconnected=off
  wires:
  Minus/1 -> Mux/3
  Minus2/1 -> Mux/2
  Minus1/1 -> Mux/1
  Gain/1 -> Q/1
  Sum of Elements1/1 -> Gain/1
  Product1/1 -> Sum of Elements1/1
  Mux/1 -> Product1/2
  Demux/3 -> Minus1/2, Minus2/1
  Demux/2 -> Minus/2, Minus1/1
  Demux/1 -> Minus/1, Minus2/2
  Sum of Elements/1 -> P/1
  Product/1 -> Sum of Elements/1
  Iabc/1 -> Product/2, Product1/1
  Vabc/1 -> Product/1, Demux/1

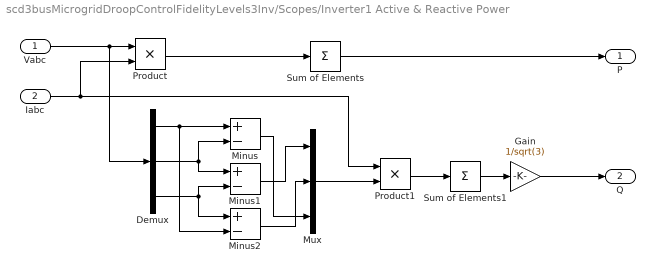
== system scd3busMicrogridDroopControlFidelityLevels3Inv/Scopes/Inverter1 Active & Reactive Power ==
  Vabc : Inport
  Iabc : Inport  Port=2
  Demux : Demux  Outputs=3
  Gain : Gain  Gain=1/sqrt(3)
  Minus : Sum  Inputs=+-
  Minus1 : Sum  Inputs=+-
  Minus2 : Sum  Inputs=+-
  Mux : Mux  Inputs=3
  Product : Product
  Product1 : Product
  Sum of Elements : Sum  Inputs=+
  Sum of Elements1 : Sum  Inputs=+
  P : Outport  VectorParamsAs1DForOutWhenUnconnected=off
  Q : Outport  Port=2  VectorParamsAs1DForOutWhenUnconnected=off
  wires:
  Vabc/1 -> Demux/1, Product/1
  Iabc/1 -> Product1/1, Product/2
  Product/1 -> Sum of Elements/1
  Sum of Elements/1 -> P/1
  Demux/1 -> Minus2/2, Minus/1
  Demux/2 -> Minus1/1, Minus/2
  Demux/3 -> Minus2/1, Minus1/2
  Mux/1 -> Product1/2
  Product1/1 -> Sum of Elements1/1
  Sum of Elements1/1 -> Gain/1
  Gain/1 -> Q/1
  Minus1/1 -> Mux/1
  Minus2/1 -> Mux/2
  Minus/1 -> Mux/3

== system scd3busMicrogridDroopControlFidelityLevels3Inv/Inverter 1/Droop Controller Inverter1/DQ Voltage Reference ==
  freq_cmd : Inport
  V_cmd : Inport  Port=2
  Gain : Gain  Gain=2*pi
  Integrator : Integrator
  Product : Product
  Product1 : Product
  Trigonometric Function : Trigonometry
  Trigonometric Function1 : Trigonometry  Operator=cos
  Vd_ref : Outport
  Vq_ref : Outport  Port=2
  wires:
  Gain/1 -> Integrator/1
  Trigonometric Function1/1 -> Product1/2
  freq_cmd/1 -> Gain/1
  Integrator/1 -> Trigonometric Function1/1, Trigonometric Function/1
  V_cmd/1 -> Product1/1, Product/2
  Trigonometric Function/1 -> Product/1
  Product1/1 -> Vd_ref/1  "Vd_ref"
  Product/1 -> Vq_ref/1  "Vq_ref"

== system scd3busMicrogridDroopControlFidelityLevels3Inv/Inverter 1/Inverter 1/Averaged Inverter ==
  Averaged Inverter : ee_lib/Semiconductors & Converters/Converters/Converter (Three-Phase)  port_option=ee.enum.threePhasePort.expanded  fidelity_option=ee.enum.converters.fidelity.detailed  device_type=ee.enum.converters.switchingdevice.averaged  showThermalPort=false  K=0  Vth=0.5 V  Vgt=1e-3 V  Vgt_off=-1 V  Ih=1 A  Vf=0.8 V  Ron=1.0000e-03 Ohm  Rds=0.001 Ohm  Goff=2.0000e-04 1/Ohm  Eon_scalar=22.86e-3 J  Eoff_scalar=17.14e-3 J  Eoff_natural_commutation=10e-3 J  Voff=300 V  Iout_scalar=600 A  onCurrentMeasDelay=0 s  useCurrentFromPreviousCycle=false  useVoltageFromPreviousCycle=false  diode_param=ee.enum.converters.protectiondiode.nodynamics  diode_Vf=0.8 V  diode_Ron=0.001 Ohm  diode_Goff=1e-5 1/Ohm  diode_C=50 nF  diode_iRM=-235 A  diode_iF=300 A  diode_idot=-50 A/us  diode_trr_param=ee.enum.converters.diodetrr.trr_factor  diode_trr_factor=3  diode_trr=15 us  diode_Qrr=1.5e+3 s*uA  diode_rec_loss_model=ee.enum.diode.reverseRecoveryModel.fixed  diode_ErecVal=0 J  diode_scaleWithIandV=false  diode_ErecMat=zeros(2, 3) J  diode_TjrecVec=[298.15, 398.15] K  diode_IfrecVec=[.1, 1, 10] A  diode_IrecVal=10 A  diode_VrecVal=10 V  diode_tFilter=1 / 1000 / 100 s  thermal_network_parameterization=ee.enum.thermalNetworkTopology.external  Rth=[.08, .5] K/W  Rth_Cauer=[.08, .1, .5] K/W  Rth_Foster=[.08, .14, .22, .16] K/W  thermal_mass_parameterization=ee.enum.thermalNetwork.timeconstant  thermal_mass=[.01, .5] J/K  thermal_mass_Cauer=[.01, .1, .5] J/K  thermal_mass_Foster=[.001, .005, .05, .5] J/K  thermal_time_constant=[.001, .2] s  thermal_time_constant_Cauer=[.001, .1, .2] s  thermal_time_constant_Foster=[7e-05, .0007, .01, .08] s  thermal_mass_initial_temperatures=[25, 25] degC  thermal_mass_initial_temperatures_Cauer=[25, 25, 25] degC  junction_thermal_mass=0.01 J/K  Tvec_initial_Foster=[25, 25, 25, 25] degC  snubber_type=ee.enum.converters.snubber.exclude  Cs=1e-7 F  Rs=0.1 Ohm  Vce_loss=[0, 150, 300] V
      settings: InternalSimscapePortConfiguration="{\"Bottom\":[],\"Left\":[{\"id\":\"G\",\"label\":\"G\",\"type\":\"foundation.electrical.twelve_phase\"},{\"id\":\"a\",\"label\":\"a\",\"type\":\"foundation.electrical.electrical\"},{\"id\":\"b\",\"label\":\"b\",\"type\":\"foundation.electrical.electrical\"},{\"id\":\"c\",\"label\":\"c\",\"type\":\"foundation.electrical.electrical\"}],\"Right\":[{\"id\":\"p\",\"label\":\"+\",\"type\":\"foundation.electrical.electrical\"},{\"id\":\"n\",\"label\":\"-\",\"type\":\"foundation.electrical.electrical\"}],\"Top\":[]}"
  + : PMIOPort  Side=Right
  G : PMIOPort  Port=2  Side=Left
  a : PMIOPort  Port=3  Side=Left
  b : PMIOPort  Port=4  Side=Left
  - : PMIOPort  Port=5  Side=Right
  c : PMIOPort  Port=6  Side=Left
  connections:
  c/RConn1 -- Averaged Inverter/LConn4
  a/RConn1 -- Averaged Inverter/LConn2
  G/RConn1 -- Averaged Inverter/LConn1
  -/RConn1 -- Averaged Inverter/RConn2
  b/RConn1 -- Averaged Inverter/LConn3
  +/RConn1 -- Averaged Inverter/RConn1

== system scd3busMicrogridDroopControlFidelityLevels3Inv/Inverter 1/Inverter 1/IGBT Inverter ==
  IGBT Inverter : ee_lib/Semiconductors & Converters/Converters/Converter (Three-Phase)  port_option=ee.enum.threePhasePort.expanded  fidelity_option=ee.enum.converters.fidelity.detailed  device_type=ee.enum.converters.switchingdevice.igbt  showThermalPort=false  K=0  Vth=0.5 V  Vgt=1e-3 V  Vgt_off=-1 V  Ih=1 A  Vf=0.8 V  Ron=1.0000e-03 Ohm  Rds=0.001 Ohm  Goff=2.0000e-04 1/Ohm  Eon_scalar=22.86e-3 J  Eoff_scalar=17.14e-3 J  Eoff_natural_commutation=10e-3 J  Voff=300 V  Iout_scalar=600 A  onCurrentMeasDelay=0 s  useCurrentFromPreviousCycle=false  useVoltageFromPreviousCycle=false  diode_param=ee.enum.converters.protectiondiode.nodynamics  diode_Vf=0.8 V  diode_Ron=0.001 Ohm  diode_Goff=1e-5 1/Ohm  diode_C=50 nF  diode_iRM=-235 A  diode_iF=300 A  diode_idot=-50 A/us  diode_trr_param=ee.enum.converters.diodetrr.trr_factor  diode_trr_factor=3  diode_trr=15 us  diode_Qrr=1.5e+3 s*uA  diode_rec_loss_model=ee.enum.diode.reverseRecoveryModel.fixed  diode_ErecVal=0 J  diode_scaleWithIandV=false  diode_ErecMat=zeros(2, 3) J  diode_TjrecVec=[298.15, 398.15] K  diode_IfrecVec=[.1, 1, 10] A  diode_IrecVal=10 A  diode_VrecVal=10 V  diode_tFilter=1 / 1000 / 100 s  thermal_network_parameterization=ee.enum.thermalNetworkTopology.external  Rth=[.08, .5] K/W  Rth_Cauer=[.08, .1, .5] K/W  Rth_Foster=[.08, .14, .22, .16] K/W  thermal_mass_parameterization=ee.enum.thermalNetwork.timeconstant  thermal_mass=[.01, .5] J/K  thermal_mass_Cauer=[.01, .1, .5] J/K  thermal_mass_Foster=[.001, .005, .05, .5] J/K  thermal_time_constant=[.001, .2] s  thermal_time_constant_Cauer=[.001, .1, .2] s  thermal_time_constant_Foster=[7e-05, .0007, .01, .08] s  thermal_mass_initial_temperatures=[25, 25] degC  thermal_mass_initial_temperatures_Cauer=[25, 25, 25] degC  junction_thermal_mass=0.01 J/K  Tvec_initial_Foster=[25, 25, 25, 25] degC  snubber_type=ee.enum.converters.snubber.exclude  Cs=1e-7 F  Rs=0.1 Ohm  Vce_loss=[0, 150, 300] V
      settings: InternalSimscapePortConfiguration="{\"Bottom\":[],\"Left\":[{\"id\":\"G\",\"label\":\"G\",\"type\":\"foundation.electrical.twelve_phase\"},{\"id\":\"a\",\"label\":\"a\",\"type\":\"foundation.electrical.electrical\"},{\"id\":\"b\",\"label\":\"b\",\"type\":\"foundation.electrical.electrical\"},{\"id\":\"c\",\"label\":\"c\",\"type\":\"foundation.electrical.electrical\"}],\"Right\":[{\"id\":\"p\",\"label\":\"+\",\"type\":\"foundation.electrical.electrical\"},{\"id\":\"n\",\"label\":\"-\",\"type\":\"foundation.electrical.electrical\"}],\"Top\":[]}"
  + : PMIOPort  Side=Right
  G : PMIOPort  Port=2  Side=Left
  a : PMIOPort  Port=3  Side=Left
  b : PMIOPort  Port=4  Side=Left
  - : PMIOPort  Port=5  Side=Right
  c : PMIOPort  Port=6  Side=Left
  connections:
  +/RConn1 -- IGBT Inverter/RConn1
  b/RConn1 -- IGBT Inverter/LConn3
  -/RConn1 -- IGBT Inverter/RConn2
  G/RConn1 -- IGBT Inverter/LConn1
  a/RConn1 -- IGBT Inverter/LConn2
  c/RConn1 -- IGBT Inverter/LConn4

== system scd3busMicrogridDroopControlFidelityLevels3Inv/Inverter 1/Solar1/MPPT Algorithm ==
  I : Inport
  V : Inport  Port=2
  D_init : Constant  Value=0.25
  D_max : Constant  Value=0.4
  D_min : Constant  Value=0.1
  Delta_D : Constant  Value=0.001
  MPPT Algorithm : MATLAB Function  SystemSampleTime=Ts
  Unit Delay : UnitDelay  InitialCondition=0.2  SampleTime=0.01
  Vector Concatenate : Concatenate  NumInputs=4
  duty_cycle : Outport
  wires:
  V/1 -> MPPT Algorithm/2(V)
  Vector Concatenate/1 -> MPPT Algorithm/1(Param)
  D_max/1 -> Vector Concatenate/2
  D_init/1 -> Vector Concatenate/1
  D_min/1 -> Vector Concatenate/3
  MPPT Algorithm/1(D) -> Unit Delay/1
  Delta_D/1 -> Vector Concatenate/4
  I/1 -> MPPT Algorithm/3(I)
  Unit Delay/1 -> duty_cycle/1

== system scd3busMicrogridDroopControlFidelityLevels3Inv/Inverter 1/Solar1/Sensing Current ==
  Current Sensor : fl_lib/Electrical/Electrical Sensors/Current Sensor
  PS-Simulink/I : nesl_utility/PS-Simulink Converter  PhysicalDomain=network_engine_domain  SubClassName=ps_output  LeftPortType=input  RightPortType=output  PseudoPeriodic=off  Frequencies=[]  VectorFormat=1-D array  Unit=1  AffineConversion=off
  + : PMIOPort  Side=Left
  - : PMIOPort  Port=2  Side=Right
  I : Outport
  wires:
  PS-Simulink/I/1 -> I/1
  connections:
  -/RConn1 -- Current Sensor/RConn2
  Current Sensor/LConn1 -- +/RConn1
  Current Sensor/RConn1 -- PS-Simulink/I/LConn1

== system scd3busMicrogridDroopControlFidelityLevels3Inv/Inverter 1/Solar1/sensing voltage ==
  PS-Simulink Converter : nesl_utility/PS-Simulink Converter  PhysicalDomain=network_engine_domain  SubClassName=ps_output  LeftPortType=input  RightPortType=output  PseudoPeriodic=off  Frequencies=[]  VectorFormat=1-D array  Unit=inherit  AffineConversion=off
  Voltage Sensor : fl_lib/Electrical/Electrical Sensors/Voltage Sensor
  + : PMIOPort  Side=Left
  - : PMIOPort  Port=2  Side=Right
  V : Outport
  wires:
  PS-Simulink Converter/1 -> V/1
  connections:
  Voltage Sensor/LConn1 -- +/RConn1
  Voltage Sensor/RConn2 -- -/RConn1
  Voltage Sensor/RConn1 -- PS-Simulink Converter/LConn1

== system scd3busMicrogridDroopControlFidelityLevels3Inv/Inverter 2/Droop Controller Inverter2/DQ Voltage Reference ==
  freq_cmd : Inport
  V_cmd : Inport  Port=2
  Gain : Gain  Gain=2*pi
  Integrator : Integrator
  Product : Product
  Product1 : Product
  Trigonometric Function : Trigonometry
  Trigonometric Function1 : Trigonometry  Operator=cos
  Vd_ref : Outport
  Vq_ref : Outport  Port=2
  wires:
  Product/1 -> Vq_ref/1  "Vq_ref"
  Product1/1 -> Vd_ref/1  "Vd_ref"
  Trigonometric Function/1 -> Product/1
  V_cmd/1 -> Product/2, Product1/1
  Integrator/1 -> Trigonometric Function/1, Trigonometric Function1/1
  freq_cmd/1 -> Gain/1
  Trigonometric Function1/1 -> Product1/2
  Gain/1 -> Integrator/1

== system scd3busMicrogridDroopControlFidelityLevels3Inv/Inverter 2/Inverter 2/Averaged Inverter ==
  Averaged Inverter : ee_lib/Semiconductors & Converters/Converters/Converter (Three-Phase)  port_option=ee.enum.threePhasePort.expanded  fidelity_option=ee.enum.converters.fidelity.detailed  device_type=ee.enum.converters.switchingdevice.averaged  showThermalPort=false  K=0  Vth=0.5 V  Vgt=1e-3 V  Vgt_off=-1 V  Ih=1 A  Vf=0.8 V  Ron=1.0000e-03 Ohm  Rds=0.001 Ohm  Goff=2.0000e-04 1/Ohm  Eon_scalar=22.86e-3 J  Eoff_scalar=17.14e-3 J  Eoff_natural_commutation=10e-3 J  Voff=300 V  Iout_scalar=600 A  onCurrentMeasDelay=0 s  useCurrentFromPreviousCycle=false  useVoltageFromPreviousCycle=false  diode_param=ee.enum.converters.protectiondiode.nodynamics  diode_Vf=0.8 V  diode_Ron=0.001 Ohm  diode_Goff=1e-5 1/Ohm  diode_C=50 nF  diode_iRM=-235 A  diode_iF=300 A  diode_idot=-50 A/us  diode_trr_param=ee.enum.converters.diodetrr.trr_factor  diode_trr_factor=3  diode_trr=15 us  diode_Qrr=1.5e+3 s*uA  diode_rec_loss_model=ee.enum.diode.reverseRecoveryModel.fixed  diode_ErecVal=0 J  diode_scaleWithIandV=false  diode_ErecMat=zeros(2, 3) J  diode_TjrecVec=[298.15, 398.15] K  diode_IfrecVec=[.1, 1, 10] A  diode_IrecVal=10 A  diode_VrecVal=10 V  diode_tFilter=1 / 1000 / 100 s  thermal_network_parameterization=ee.enum.thermalNetworkTopology.external  Rth=[.08, .5] K/W  Rth_Cauer=[.08, .1, .5] K/W  Rth_Foster=[.08, .14, .22, .16] K/W  thermal_mass_parameterization=ee.enum.thermalNetwork.timeconstant  thermal_mass=[.01, .5] J/K  thermal_mass_Cauer=[.01, .1, .5] J/K  thermal_mass_Foster=[.001, .005, .05, .5] J/K  thermal_time_constant=[.001, .2] s  thermal_time_constant_Cauer=[.001, .1, .2] s  thermal_time_constant_Foster=[7e-05, .0007, .01, .08] s  thermal_mass_initial_temperatures=[25, 25] degC  thermal_mass_initial_temperatures_Cauer=[25, 25, 25] degC  junction_thermal_mass=0.01 J/K  Tvec_initial_Foster=[25, 25, 25, 25] degC  snubber_type=ee.enum.converters.snubber.exclude  Cs=1e-7 F  Rs=0.1 Ohm  Vce_loss=[0, 150, 300] V
      settings: InternalSimscapePortConfiguration="{\"Bottom\":[],\"Left\":[{\"id\":\"G\",\"label\":\"G\",\"type\":\"foundation.electrical.twelve_phase\"},{\"id\":\"a\",\"label\":\"a\",\"type\":\"foundation.electrical.electrical\"},{\"id\":\"b\",\"label\":\"b\",\"type\":\"foundation.electrical.electrical\"},{\"id\":\"c\",\"label\":\"c\",\"type\":\"foundation.electrical.electrical\"}],\"Right\":[{\"id\":\"p\",\"label\":\"+\",\"type\":\"foundation.electrical.electrical\"},{\"id\":\"n\",\"label\":\"-\",\"type\":\"foundation.electrical.electrical\"}],\"Top\":[]}"
  + : PMIOPort  Side=Right
  G : PMIOPort  Port=2  Side=Left
  a : PMIOPort  Port=3  Side=Left
  b : PMIOPort  Port=4  Side=Left
  - : PMIOPort  Port=5  Side=Right
  c : PMIOPort  Port=6  Side=Left
  connections:
  +/RConn1 -- Averaged Inverter/RConn1
  b/RConn1 -- Averaged Inverter/LConn3
  -/RConn1 -- Averaged Inverter/RConn2
  G/RConn1 -- Averaged Inverter/LConn1
  a/RConn1 -- Averaged Inverter/LConn2
  c/RConn1 -- Averaged Inverter/LConn4

== system scd3busMicrogridDroopControlFidelityLevels3Inv/Inverter 2/Inverter 2/IGBT Inverter ==
  IGBT Inverter : ee_lib/Semiconductors & Converters/Converters/Converter (Three-Phase)  port_option=ee.enum.threePhasePort.expanded  fidelity_option=ee.enum.converters.fidelity.detailed  device_type=ee.enum.converters.switchingdevice.igbt  showThermalPort=false  K=0  Vth=0.5 V  Vgt=1e-3 V  Vgt_off=-1 V  Ih=1 A  Vf=0.8 V  Ron=1.0000e-03 Ohm  Rds=0.001 Ohm  Goff=2.0000e-04 1/Ohm  Eon_scalar=22.86e-3 J  Eoff_scalar=17.14e-3 J  Eoff_natural_commutation=10e-3 J  Voff=300 V  Iout_scalar=600 A  onCurrentMeasDelay=0 s  useCurrentFromPreviousCycle=false  useVoltageFromPreviousCycle=false  diode_param=ee.enum.converters.protectiondiode.nodynamics  diode_Vf=0.8 V  diode_Ron=0.001 Ohm  diode_Goff=1e-5 1/Ohm  diode_C=50 nF  diode_iRM=-235 A  diode_iF=300 A  diode_idot=-50 A/us  diode_trr_param=ee.enum.converters.diodetrr.trr_factor  diode_trr_factor=3  diode_trr=15 us  diode_Qrr=1.5e+3 s*uA  diode_rec_loss_model=ee.enum.diode.reverseRecoveryModel.fixed  diode_ErecVal=0 J  diode_scaleWithIandV=false  diode_ErecMat=zeros(2, 3) J  diode_TjrecVec=[298.15, 398.15] K  diode_IfrecVec=[.1, 1, 10] A  diode_IrecVal=10 A  diode_VrecVal=10 V  diode_tFilter=1 / 1000 / 100 s  thermal_network_parameterization=ee.enum.thermalNetworkTopology.external  Rth=[.08, .5] K/W  Rth_Cauer=[.08, .1, .5] K/W  Rth_Foster=[.08, .14, .22, .16] K/W  thermal_mass_parameterization=ee.enum.thermalNetwork.timeconstant  thermal_mass=[.01, .5] J/K  thermal_mass_Cauer=[.01, .1, .5] J/K  thermal_mass_Foster=[.001, .005, .05, .5] J/K  thermal_time_constant=[.001, .2] s  thermal_time_constant_Cauer=[.001, .1, .2] s  thermal_time_constant_Foster=[7e-05, .0007, .01, .08] s  thermal_mass_initial_temperatures=[25, 25] degC  thermal_mass_initial_temperatures_Cauer=[25, 25, 25] degC  junction_thermal_mass=0.01 J/K  Tvec_initial_Foster=[25, 25, 25, 25] degC  snubber_type=ee.enum.converters.snubber.exclude  Cs=1e-7 F  Rs=0.1 Ohm  Vce_loss=[0, 150, 300] V
      settings: InternalSimscapePortConfiguration="{\"Bottom\":[],\"Left\":[{\"id\":\"G\",\"label\":\"G\",\"type\":\"foundation.electrical.twelve_phase\"},{\"id\":\"a\",\"label\":\"a\",\"type\":\"foundation.electrical.electrical\"},{\"id\":\"b\",\"label\":\"b\",\"type\":\"foundation.electrical.electrical\"},{\"id\":\"c\",\"label\":\"c\",\"type\":\"foundation.electrical.electrical\"}],\"Right\":[{\"id\":\"p\",\"label\":\"+\",\"type\":\"foundation.electrical.electrical\"},{\"id\":\"n\",\"label\":\"-\",\"type\":\"foundation.electrical.electrical\"}],\"Top\":[]}"
  + : PMIOPort  Side=Right
  G : PMIOPort  Port=2  Side=Left
  a : PMIOPort  Port=3  Side=Left
  b : PMIOPort  Port=4  Side=Left
  - : PMIOPort  Port=5  Side=Right
  c : PMIOPort  Port=6  Side=Left
  connections:
  c/RConn1 -- IGBT Inverter/LConn4
  a/RConn1 -- IGBT Inverter/LConn2
  G/RConn1 -- IGBT Inverter/LConn1
  -/RConn1 -- IGBT Inverter/RConn2
  b/RConn1 -- IGBT Inverter/LConn3
  +/RConn1 -- IGBT Inverter/RConn1
